simulink model "GraphFun1"  (Simulink 6.0)
settings: Solver=FixedStepDiscrete  StartTime=0.0  StopTime=inf  RelTol=1e-3
settings Model: Creator=scaife  LastModifiedBy=scaife  ExtModeAutoUpdateStatusClock=off
settings DebuggingCC: AlgebraicLoopMsg=error

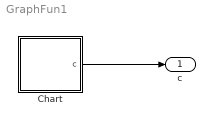
== system GraphFun1 ==
  Chart : Stateflow chart
  c : Outport
  wires:
  Chart/1(c) -> c/1

== stateflow chart Chart ==
  state A/
    en:a=3,b=4
  state B/
    en:a=5,b=12
  state z=f(x,y) [function]
    (default) -> (junction 6) : {z=sqrt(x*x+y*y);}
  (default) -> A
  A -> B : {c=f(a,b)}
  B -> A : {c=f(a,b)}
  data: x function_input double; y function_input double; z function_output double; a local double; b local double; c output double
